simulink subsystem "acceleration_car"  (R2025b)
settings: Solver=VariableStepAuto  StartTime=0.0  StopTime=10.0  RelTol=1e-3
settings Model: Creator=sanborkl  LastModifiedBy=sanborkl

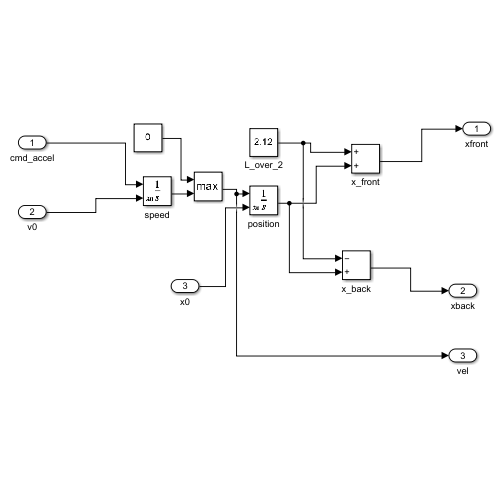
[thumbnail: Simulink's stored preview of the top-level diagram]
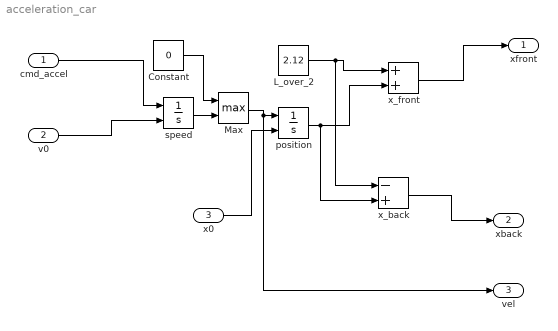
== system acceleration_car ==
  cmd_accel : Inport
  v0 : Inport  Port=2
  x0 : Inport  Port=3
  Constant : Constant  Value=0
  L_over_2 : Constant  Value=2.12
  Max : MinMax  Function=max  Inputs=2
  position : Integrator  InitialConditionSource=external
  speed : Integrator  InitialConditionSource=external
  x_back : Sum  Inputs=-+
  x_front : Sum
  xfront : Outport
  xback : Outport  Port=2
  vel : Outport  Port=3
  wires:
  speed/1 -> Max/2
  position/1 -> x_front/2, x_back/2
  x0/1 -> position/2
  v0/1 -> speed/2
  cmd_accel/1 -> speed/1
  Constant/1 -> Max/1
  L_over_2/1 -> x_front/1, x_back/1
  x_back/1 -> xback/1
  Max/1 -> position/1, vel/1
  x_front/1 -> xfront/1
